simulink model "twowheeledrobot"  (R2021a)
settings: Solver=ode4  StartTime=0  StopTime=40  FixedStep=1e-2  RelTol=1e-3  AbsTol=1e-6
settings Model: ExtModeTrigMode=oneshot  ExtModeArmWhenConnect=off  Creator=jerome  LastModifiedBy=davidrico
settings SolverCC: AutoScaleAbsTol=off  AlgebraicLoopSolver=TrustRegion
settings DataIOCC: SaveFormat=Array  SignalLoggingSaveFormat=ModelDataLogs  ReturnWorkspaceOutputs=off
settings OptimizationCC: BlockReduction=off  BooleanDataType=off  ExpressionDepthLimit=2147483647  InitFltsAndDblsToZero=on  LifeSpan=inf
settings DebuggingCC: SaveWithParameterizedLinksMsg=none  UnderspecifiedInitializationDetection=Classic  MergeDetectMultiDrivingBlocksExec=none  SignalResolutionControl=TryResolveAllWithWarning  MultiTaskDSMMsg=warning  MultiTaskCondExecSysMsg=none  FcnCallInpInsideContextMsg=warning  StateNameClashWarn=warning  SFUnexpectedBacktrackingDiag=warning  SFNoUnconditionalDefaultTransitionDiag=warning  SFExecutionAtInitializationDiag=none  SFMachineParentedDataDiag=warning  ArithmeticOperatorsInVariantConditions=warning
settings HardwareCC: ProdBitPerPointer=32  ProdBitPerSizeT=32  ProdBitPerPtrDiffT=32  ProdLargestAtomicFloat=None  ProdIntDivRoundTo=Undefined  ProdEndianess=Unspecified  ProdWordSize=32  ProdHWDeviceType=32-bit Generic  TargetUnknown=on
settings ModelReferenceCC: PropagateSignalLabelsOutOfModel=off
settings SFSimCC: SimUseLocalCustomCode=off  CustomCodeUndefinedFunction=UseInterfaceOnly
settings RTWCC: RTWUseLocalCustomCode=off
settings CodeAppCC: StateflowObjectComments=on
settings GRTTargetCC: TargetFcnLib=ansi_tfl_tmw.mat  TargetLangStandard=C89/C90 (ANSI)  ModelReferenceCompliant=off  CombineOutputUpdateFcns=off  MatFileLogging=off  GRTInterface=on
settings ConfigComp: CovMetricSettings=dw  CovSaveCumulativeToWorkspaceVar=on  CovSaveSingleToWorkspaceVar=on  CovExternalEMLEnable=off

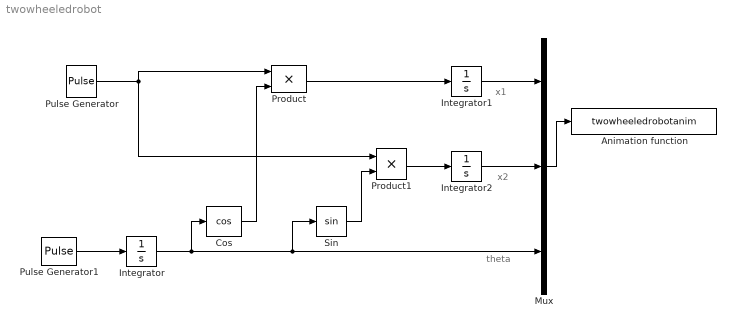
== system twowheeledrobot ==
  note: theta
  note: x2
  note: x1
  Animation function : S-Function  FunctionName=twowheeledrobotanim  SFunctionDeploymentMode=off  EnableBusSupport=off
  Cos : Trigonometry  Operator=cos
  Integrator : Integrator
  Integrator1 : Integrator  UpperSaturationLimit=1
  Integrator2 : Integrator  UpperSaturationLimit=1
  Mux : Mux  Inputs=3
  Product : Product
  Product1 : Product
  Pulse Generator : DiscretePulseGenerator  PulseType=Time based  Period=10  PulseWidth=50
  Pulse Generator1 : DiscretePulseGenerator  PulseType=Time based  Amplitude=pi/2  Period=10  PulseWidth=50  PhaseDelay=5.0
  Sin : Trigonometry
  wires:
  Mux/1 -> Animation function/1
  Cos/1 -> Product/2
  Sin/1 -> Product1/2
  Pulse Generator1/1 -> Integrator/1
  Pulse Generator/1 -> Product1/1, Product/1
  Integrator1/1 -> Mux/1
  Product/1 -> Integrator1/1
  Product1/1 -> Integrator2/1
  Integrator2/1 -> Mux/2
  Integrator/1 -> Cos/1, Mux/3, Sin/1
